simulink model "FunctionalArchitectureProj"  (R2023b)
settings: Solver=VariableStepAuto  StartTime=0.0  StopTime=10.0  RelTol=1e-3
(part 2 of 3)

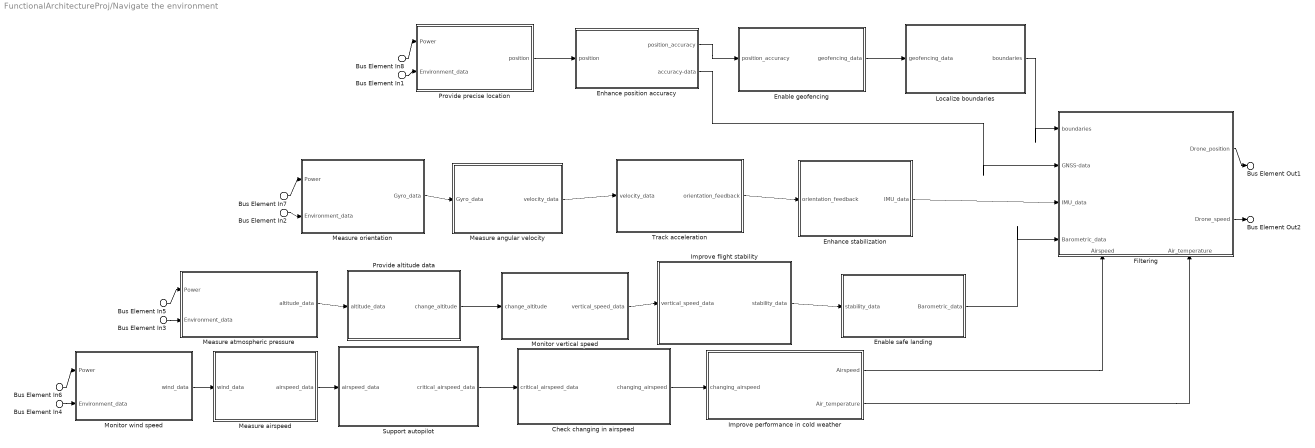
== system FunctionalArchitectureProj/Navigate the environment ==
  Bus Element In{1..4} (4 alike) : Inport  PortName=Environment_data
  Bus Element In{5..8} (4 alike) : Inport  Port=2  PortName=Power
  Check changing in airspeed : Subsystem
      settings: PortSchema="{\"entries\":[{\"content\":{\"headerSize\":26,\"margin\":15,\"minimumSpacing\":25,\"sides\":[{\"content\":{\"connectorIds\":[\"In1\"]},\"type\":\"ConnectorPlacement.EquallySpacedRectSide\",\"uuid\":\"522b493f-2ddf-45ff-a295-a4a6ad43d3e9\"},{\"content\":{\"connectorIds\":[\"Out1\"],\"side\":\"RIGHT\"},\"type\":\"ConnectorPlacement.EquallySpacedRectSide\",\"uuid\":\"9f08b077-98af-4d6e-858b-0cb586e18451\"},{\"content\":{\"side\":\"TOP\"},\"type\":\"ConnectorPlacement.EquallySpacedRectSide\",\"uuid\":\"7ff6f721-17eb-4e7e-8b3a-e93639631da6\"}]},\"type\":\"ConnectorPlacement.EquallySpacedConnector\",\"uuid\":\"bde844eb-2873-40a7-848c-24f407987c7c\"}],\"packageUris\":[\"http://schema.mathworks.com/mf0/Connector/R2020b\"],\"version\":\"1.0\"}"
  Enable geofencing : Subsystem
      settings: PortSchema="{\"entries\":[{\"content\":{\"headerSize\":26,\"margin\":15,\"minimumSpacing\":25,\"sides\":[{\"content\":{\"connectorIds\":[\"In1\"]},\"type\":\"ConnectorPlacement.EquallySpacedRectSide\",\"uuid\":\"522b493f-2ddf-45ff-a295-a4a6ad43d3e9\"},{\"content\":{\"connectorIds\":[\"Out1\"],\"side\":\"RIGHT\"},\"type\":\"ConnectorPlacement.EquallySpacedRectSide\",\"uuid\":\"9f08b077-98af-4d6e-858b-0cb586e18451\"},{\"content\":{\"side\":\"TOP\"},\"type\":\"ConnectorPlacement.EquallySpacedRectSide\",\"uuid\":\"7ff6f721-17eb-4e7e-8b3a-e93639631da6\"}]},\"type\":\"ConnectorPlacement.EquallySpacedConnector\",\"uuid\":\"bde844eb-2873-40a7-848c-24f407987c7c\"}],\"packageUris\":[\"http://schema.mathworks.com/mf0/Connector/R2020b\"],\"version\":\"1.0\"}"
  Enable safe landing : Subsystem
      settings: PortSchema="{\"entries\":[{\"content\":{\"headerSize\":26,\"margin\":15,\"minimumSpacing\":25,\"sides\":[{\"content\":{\"connectorIds\":[\"In1\"]},\"type\":\"ConnectorPlacement.EquallySpacedRectSide\",\"uuid\":\"522b493f-2ddf-45ff-a295-a4a6ad43d3e9\"},{\"content\":{\"connectorIds\":[\"Out1\"],\"side\":\"RIGHT\"},\"type\":\"ConnectorPlacement.EquallySpacedRectSide\",\"uuid\":\"9f08b077-98af-4d6e-858b-0cb586e18451\"},{\"content\":{\"side\":\"TOP\"},\"type\":\"ConnectorPlacement.EquallySpacedRectSide\",\"uuid\":\"7ff6f721-17eb-4e7e-8b3a-e93639631da6\"},{\"content\":{\"side\":\"BOTTOM\"},\"type\":\"ConnectorPlacement.EquallySpacedRectSide\",\"uuid\":\"7f58067e-8efa-428a-9e32-f5196a2d2b76\"}]},\"type\":\"ConnectorPlacement.EquallySpacedConnector\",\"uuid\":\"bde844eb-2873-40a7-848c-24f407987c7c\"}],\"packageUris\":[\"http://schema.mathworks.com/mf0/Connector/R2020b\"],\"version\":\"1.0\"}"
  Enhance position accuracy : Subsystem
      settings: PortSchema="{\"entries\":[{\"content\":{\"headerSize\":26,\"margin\":15,\"minimumSpacing\":25,\"sides\":[{\"content\":{\"connectorIds\":[\"In1\"]},\"type\":\"ConnectorPlacement.EquallySpacedRectSide\",\"uuid\":\"522b493f-2ddf-45ff-a295-a4a6ad43d3e9\"},{\"content\":{\"connectorIds\":[\"Out1\",\"Out2\"],\"side\":\"RIGHT\"},\"type\":\"ConnectorPlacement.EquallySpacedRectSide\",\"uuid\":\"9f08b077-98af-4d6e-858b-0cb586e18451\"},{\"content\":{\"side\":\"TOP\"},\"type\":\"ConnectorPlacement.EquallySpacedRectSide\",\"uuid\":\"7ff6f721-17eb-4e7e-8b3a-e93639631da6\"}]},\"type\":\"ConnectorPlacement.EquallySpacedConnector\",\"uuid\":\"bde844eb-2873-40a7-848c-24f407987c7c\"}],\"packageUris\":[\"http://schema.mathworks.com/mf0/Connector/R2020b\"],\"version\":\"1.0\"}"
  "Enhance stabilization " : Subsystem
      settings: PortSchema="{\"entries\":[{\"content\":{\"headerSize\":26,\"margin\":15,\"minimumSpacing\":25,\"sides\":[{\"content\":{\"connectorIds\":[\"In1\"]},\"type\":\"ConnectorPlacement.EquallySpacedRectSide\",\"uuid\":\"522b493f-2ddf-45ff-a295-a4a6ad43d3e9\"},{\"content\":{\"connectorIds\":[\"Out1\"],\"side\":\"RIGHT\"},\"type\":\"ConnectorPlacement.EquallySpacedRectSide\",\"uuid\":\"9f08b077-98af-4d6e-858b-0cb586e18451\"},{\"content\":{\"side\":\"TOP\"},\"type\":\"ConnectorPlacement.EquallySpacedRectSide\",\"uuid\":\"7ff6f721-17eb-4e7e-8b3a-e93639631da6\"}]},\"type\":\"ConnectorPlacement.EquallySpacedConnector\",\"uuid\":\"bde844eb-2873-40a7-848c-24f407987c7c\"}],\"packageUris\":[\"http://schema.mathworks.com/mf0/Connector/R2020b\"],\"version\":\"1.0\"}"
  Filtering : Subsystem
      settings: PortSchema="{\"entries\":[{\"content\":{\"headerSize\":26,\"margin\":15,\"minimumSpacing\":25,\"sides\":[{\"content\":{\"connectorIds\":[\"In4\",\"In5\",\"In3\",\"In6\"]},\"type\":\"ConnectorPlacement.EquallySpacedRectSide\",\"uuid\":\"522b493f-2ddf-45ff-a295-a4a6ad43d3e9\"},{\"content\":{\"connectorIds\":[\"Out1\",\"Out2\"],\"side\":\"RIGHT\"},\"type\":\"ConnectorPlacement.EquallySpacedRectSide\",\"uuid\":\"9f08b077-98af-4d6e-858b-0cb586e18451\"},{\"content\":{\"side\":\"TOP\"},\"type\":\"ConnectorPlacement.EquallySpacedRectSide\",\"uuid\":\"7ff6f721-17eb-4e7e-8b3a-e93639631da6\"},{\"content\":{\"connectorIds\":[\"In1\",\"In2\"],\"side\":\"BOTTOM\"},\"type\":\"ConnectorPlacement.EquallySpacedRectSide\",\"uuid\":\"1c17908a-7b9e-47dd-bd3a-ac0935137312\"}]},\"type\":\"ConnectorPlacement.EquallySpacedConnector\",\"uuid\":\"bde844eb-2873-40a7-848c-24f407987c7c\"}],\"packageUris\":[\"http://schema.mathworks.com/mf0/Connector/R2020b\"],\"version\":\"1.0\"}"
  Improve flight stability : Subsystem
      settings: PortSchema="{\"entries\":[{\"content\":{\"headerSize\":26,\"margin\":15,\"minimumSpacing\":25,\"sides\":[{\"content\":{\"connectorIds\":[\"In1\"]},\"type\":\"ConnectorPlacement.EquallySpacedRectSide\",\"uuid\":\"522b493f-2ddf-45ff-a295-a4a6ad43d3e9\"},{\"content\":{\"connectorIds\":[\"Out1\"],\"side\":\"RIGHT\"},\"type\":\"ConnectorPlacement.EquallySpacedRectSide\",\"uuid\":\"9f08b077-98af-4d6e-858b-0cb586e18451\"},{\"content\":{\"side\":\"TOP\"},\"type\":\"ConnectorPlacement.EquallySpacedRectSide\",\"uuid\":\"7ff6f721-17eb-4e7e-8b3a-e93639631da6\"}]},\"type\":\"ConnectorPlacement.EquallySpacedConnector\",\"uuid\":\"bde844eb-2873-40a7-848c-24f407987c7c\"}],\"packageUris\":[\"http://schema.mathworks.com/mf0/Connector/R2020b\"],\"version\":\"1.0\"}"
  Improve performance in cold weather : Subsystem
      settings: PortSchema="{\"entries\":[{\"content\":{\"headerSize\":26,\"margin\":15,\"minimumSpacing\":25,\"sides\":[{\"content\":{\"connectorIds\":[\"In1\"]},\"type\":\"ConnectorPlacement.EquallySpacedRectSide\",\"uuid\":\"522b493f-2ddf-45ff-a295-a4a6ad43d3e9\"},{\"content\":{\"connectorIds\":[\"Out1\",\"Out2\"],\"side\":\"RIGHT\"},\"type\":\"ConnectorPlacement.EquallySpacedRectSide\",\"uuid\":\"9f08b077-98af-4d6e-858b-0cb586e18451\"},{\"content\":{\"side\":\"TOP\"},\"type\":\"ConnectorPlacement.EquallySpacedRectSide\",\"uuid\":\"7ff6f721-17eb-4e7e-8b3a-e93639631da6\"}]},\"type\":\"ConnectorPlacement.EquallySpacedConnector\",\"uuid\":\"bde844eb-2873-40a7-848c-24f407987c7c\"}],\"packageUris\":[\"http://schema.mathworks.com/mf0/Connector/R2020b\"],\"version\":\"1.0\"}"
  Localize boundaries : Subsystem
      settings: PortSchema="{\"entries\":[{\"content\":{\"headerSize\":26,\"margin\":15,\"minimumSpacing\":25,\"sides\":[{\"content\":{\"connectorIds\":[\"In1\"]},\"type\":\"ConnectorPlacement.EquallySpacedRectSide\",\"uuid\":\"522b493f-2ddf-45ff-a295-a4a6ad43d3e9\"},{\"content\":{\"connectorIds\":[\"Out1\"],\"side\":\"RIGHT\"},\"type\":\"ConnectorPlacement.EquallySpacedRectSide\",\"uuid\":\"9f08b077-98af-4d6e-858b-0cb586e18451\"},{\"content\":{\"side\":\"TOP\"},\"type\":\"ConnectorPlacement.EquallySpacedRectSide\",\"uuid\":\"7ff6f721-17eb-4e7e-8b3a-e93639631da6\"}]},\"type\":\"ConnectorPlacement.EquallySpacedConnector\",\"uuid\":\"bde844eb-2873-40a7-848c-24f407987c7c\"}],\"packageUris\":[\"http://schema.mathworks.com/mf0/Connector/R2020b\"],\"version\":\"1.0\"}"
  Measure airspeed : Subsystem
      settings: PortSchema="{\"entries\":[{\"content\":{\"headerSize\":26,\"margin\":15,\"minimumSpacing\":25,\"sides\":[{\"content\":{\"connectorIds\":[\"In1\"]},\"type\":\"ConnectorPlacement.EquallySpacedRectSide\",\"uuid\":\"522b493f-2ddf-45ff-a295-a4a6ad43d3e9\"},{\"content\":{\"connectorIds\":[\"Out1\"],\"side\":\"RIGHT\"},\"type\":\"ConnectorPlacement.EquallySpacedRectSide\",\"uuid\":\"9f08b077-98af-4d6e-858b-0cb586e18451\"},{\"content\":{\"side\":\"TOP\"},\"type\":\"ConnectorPlacement.EquallySpacedRectSide\",\"uuid\":\"7ff6f721-17eb-4e7e-8b3a-e93639631da6\"}]},\"type\":\"ConnectorPlacement.EquallySpacedConnector\",\"uuid\":\"bde844eb-2873-40a7-848c-24f407987c7c\"}],\"packageUris\":[\"http://schema.mathworks.com/mf0/Connector/R2020b\"],\"version\":\"1.0\"}"
  Measure angular velocity : Subsystem
      settings: PortSchema="{\"entries\":[{\"content\":{\"headerSize\":26,\"margin\":15,\"minimumSpacing\":25,\"sides\":[{\"content\":{\"connectorIds\":[\"In1\"]},\"type\":\"ConnectorPlacement.EquallySpacedRectSide\",\"uuid\":\"522b493f-2ddf-45ff-a295-a4a6ad43d3e9\"},{\"content\":{\"connectorIds\":[\"Out1\"],\"side\":\"RIGHT\"},\"type\":\"ConnectorPlacement.EquallySpacedRectSide\",\"uuid\":\"9f08b077-98af-4d6e-858b-0cb586e18451\"},{\"content\":{\"side\":\"TOP\"},\"type\":\"ConnectorPlacement.EquallySpacedRectSide\",\"uuid\":\"7ff6f721-17eb-4e7e-8b3a-e93639631da6\"}]},\"type\":\"ConnectorPlacement.EquallySpacedConnector\",\"uuid\":\"bde844eb-2873-40a7-848c-24f407987c7c\"}],\"packageUris\":[\"http://schema.mathworks.com/mf0/Connector/R2020b\"],\"version\":\"1.0\"}"
  Measure atmospheric pressure : Subsystem
      settings: PortSchema="{\"entries\":[{\"content\":{\"headerSize\":26,\"margin\":15,\"minimumSpacing\":25,\"sides\":[{\"content\":{\"connectorIds\":[\"In1\",\"In2\"]},\"type\":\"ConnectorPlacement.EquallySpacedRectSide\",\"uuid\":\"522b493f-2ddf-45ff-a295-a4a6ad43d3e9\"},{\"content\":{\"connectorIds\":[\"Out1\"],\"side\":\"RIGHT\"},\"type\":\"ConnectorPlacement.EquallySpacedRectSide\",\"uuid\":\"9f08b077-98af-4d6e-858b-0cb586e18451\"},{\"content\":{\"side\":\"TOP\"},\"type\":\"ConnectorPlacement.EquallySpacedRectSide\",\"uuid\":\"7ff6f721-17eb-4e7e-8b3a-e93639631da6\"}]},\"type\":\"ConnectorPlacement.EquallySpacedConnector\",\"uuid\":\"bde844eb-2873-40a7-848c-24f407987c7c\"}],\"packageUris\":[\"http://schema.mathworks.com/mf0/Connector/R2020b\"],\"version\":\"1.0\"}"
  Measure orientation : Subsystem
      settings: PortSchema="{\"entries\":[{\"content\":{\"headerSize\":26,\"margin\":15,\"minimumSpacing\":25,\"sides\":[{\"content\":{\"connectorIds\":[\"In1\",\"In2\"]},\"type\":\"ConnectorPlacement.EquallySpacedRectSide\",\"uuid\":\"522b493f-2ddf-45ff-a295-a4a6ad43d3e9\"},{\"content\":{\"connectorIds\":[\"Out1\"],\"side\":\"RIGHT\"},\"type\":\"ConnectorPlacement.EquallySpacedRectSide\",\"uuid\":\"9f08b077-98af-4d6e-858b-0cb586e18451\"},{\"content\":{\"side\":\"TOP\"},\"type\":\"ConnectorPlacement.EquallySpacedRectSide\",\"uuid\":\"7ff6f721-17eb-4e7e-8b3a-e93639631da6\"}]},\"type\":\"ConnectorPlacement.EquallySpacedConnector\",\"uuid\":\"bde844eb-2873-40a7-848c-24f407987c7c\"}],\"packageUris\":[\"http://schema.mathworks.com/mf0/Connector/R2020b\"],\"version\":\"1.0\"}"
  Monitor vertical speed : Subsystem
      settings: PortSchema="{\"entries\":[{\"content\":{\"headerSize\":26,\"margin\":15,\"minimumSpacing\":25,\"sides\":[{\"content\":{\"connectorIds\":[\"In1\"]},\"type\":\"ConnectorPlacement.EquallySpacedRectSide\",\"uuid\":\"522b493f-2ddf-45ff-a295-a4a6ad43d3e9\"},{\"content\":{\"connectorIds\":[\"Out1\"],\"side\":\"RIGHT\"},\"type\":\"ConnectorPlacement.EquallySpacedRectSide\",\"uuid\":\"9f08b077-98af-4d6e-858b-0cb586e18451\"},{\"content\":{\"side\":\"TOP\"},\"type\":\"ConnectorPlacement.EquallySpacedRectSide\",\"uuid\":\"7ff6f721-17eb-4e7e-8b3a-e93639631da6\"}]},\"type\":\"ConnectorPlacement.EquallySpacedConnector\",\"uuid\":\"bde844eb-2873-40a7-848c-24f407987c7c\"}],\"packageUris\":[\"http://schema.mathworks.com/mf0/Connector/R2020b\"],\"version\":\"1.0\"}"
  Monitor wind speed : Subsystem
      settings: PortSchema="{\"entries\":[{\"content\":{\"headerSize\":26,\"margin\":15,\"minimumSpacing\":25,\"sides\":[{\"content\":{\"connectorIds\":[\"In1\",\"In2\"]},\"type\":\"ConnectorPlacement.EquallySpacedRectSide\",\"uuid\":\"522b493f-2ddf-45ff-a295-a4a6ad43d3e9\"},{\"content\":{\"connectorIds\":[\"Out1\"],\"side\":\"RIGHT\"},\"type\":\"ConnectorPlacement.EquallySpacedRectSide\",\"uuid\":\"9f08b077-98af-4d6e-858b-0cb586e18451\"},{\"content\":{\"side\":\"TOP\"},\"type\":\"ConnectorPlacement.EquallySpacedRectSide\",\"uuid\":\"7ff6f721-17eb-4e7e-8b3a-e93639631da6\"}]},\"type\":\"ConnectorPlacement.EquallySpacedConnector\",\"uuid\":\"bde844eb-2873-40a7-848c-24f407987c7c\"}],\"packageUris\":[\"http://schema.mathworks.com/mf0/Connector/R2020b\"],\"version\":\"1.0\"}"
  Provide altitude data : Subsystem
      settings: PortSchema="{\"entries\":[{\"content\":{\"headerSize\":26,\"margin\":15,\"minimumSpacing\":25,\"sides\":[{\"content\":{\"connectorIds\":[\"In1\"]},\"type\":\"ConnectorPlacement.EquallySpacedRectSide\",\"uuid\":\"522b493f-2ddf-45ff-a295-a4a6ad43d3e9\"},{\"content\":{\"connectorIds\":[\"Out1\"],\"side\":\"RIGHT\"},\"type\":\"ConnectorPlacement.EquallySpacedRectSide\",\"uuid\":\"9f08b077-98af-4d6e-858b-0cb586e18451\"},{\"content\":{\"side\":\"TOP\"},\"type\":\"ConnectorPlacement.EquallySpacedRectSide\",\"uuid\":\"7ff6f721-17eb-4e7e-8b3a-e93639631da6\"}]},\"type\":\"ConnectorPlacement.EquallySpacedConnector\",\"uuid\":\"bde844eb-2873-40a7-848c-24f407987c7c\"}],\"packageUris\":[\"http://schema.mathworks.com/mf0/Connector/R2020b\"],\"version\":\"1.0\"}"
  Provide precise location : Subsystem
      settings: PortSchema="{\"entries\":[{\"content\":{\"headerSize\":26,\"margin\":15,\"minimumSpacing\":25,\"sides\":[{\"content\":{\"connectorIds\":[\"In1\",\"In2\"]},\"type\":\"ConnectorPlacement.EquallySpacedRectSide\",\"uuid\":\"522b493f-2ddf-45ff-a295-a4a6ad43d3e9\"},{\"content\":{\"connectorIds\":[\"Out1\"],\"side\":\"RIGHT\"},\"type\":\"ConnectorPlacement.EquallySpacedRectSide\",\"uuid\":\"9f08b077-98af-4d6e-858b-0cb586e18451\"},{\"content\":{\"side\":\"TOP\"},\"type\":\"ConnectorPlacement.EquallySpacedRectSide\",\"uuid\":\"7ff6f721-17eb-4e7e-8b3a-e93639631da6\"}]},\"type\":\"ConnectorPlacement.EquallySpacedConnector\",\"uuid\":\"bde844eb-2873-40a7-848c-24f407987c7c\"}],\"packageUris\":[\"http://schema.mathworks.com/mf0/Connector/R2020b\"],\"version\":\"1.0\"}"
  Support autopilot : Subsystem
      settings: PortSchema="{\"entries\":[{\"content\":{\"headerSize\":26,\"margin\":15,\"minimumSpacing\":25,\"sides\":[{\"content\":{\"connectorIds\":[\"In1\"]},\"type\":\"ConnectorPlacement.EquallySpacedRectSide\",\"uuid\":\"522b493f-2ddf-45ff-a295-a4a6ad43d3e9\"},{\"content\":{\"connectorIds\":[\"Out1\"],\"side\":\"RIGHT\"},\"type\":\"ConnectorPlacement.EquallySpacedRectSide\",\"uuid\":\"9f08b077-98af-4d6e-858b-0cb586e18451\"},{\"content\":{\"side\":\"TOP\"},\"type\":\"ConnectorPlacement.EquallySpacedRectSide\",\"uuid\":\"7ff6f721-17eb-4e7e-8b3a-e93639631da6\"}]},\"type\":\"ConnectorPlacement.EquallySpacedConnector\",\"uuid\":\"bde844eb-2873-40a7-848c-24f407987c7c\"}],\"packageUris\":[\"http://schema.mathworks.com/mf0/Connector/R2020b\"],\"version\":\"1.0\"}"
  Track acceleration : Subsystem
      settings: PortSchema="{\"entries\":[{\"content\":{\"headerSize\":26,\"margin\":15,\"minimumSpacing\":25,\"sides\":[{\"content\":{\"connectorIds\":[\"In1\"]},\"type\":\"ConnectorPlacement.EquallySpacedRectSide\",\"uuid\":\"522b493f-2ddf-45ff-a295-a4a6ad43d3e9\"},{\"content\":{\"connectorIds\":[\"Out1\"],\"side\":\"RIGHT\"},\"type\":\"ConnectorPlacement.EquallySpacedRectSide\",\"uuid\":\"9f08b077-98af-4d6e-858b-0cb586e18451\"},{\"content\":{\"side\":\"TOP\"},\"type\":\"ConnectorPlacement.EquallySpacedRectSide\",\"uuid\":\"7ff6f721-17eb-4e7e-8b3a-e93639631da6\"}]},\"type\":\"ConnectorPlacement.EquallySpacedConnector\",\"uuid\":\"bde844eb-2873-40a7-848c-24f407987c7c\"}],\"packageUris\":[\"http://schema.mathworks.com/mf0/Connector/R2020b\"],\"version\":\"1.0\"}"
  Bus Element Out1 : Outport  PortName=Drone_position
  Bus Element Out2 : Outport  Port=2  PortName=Drone_speed
  wires:
  Provide precise location/1(position) -> Enhance position accuracy/1(position)
  Enhance position accuracy/1(position_accuracy) -> Enable geofencing/1(position_accuracy)
  Enable geofencing/1(geofencing_data) -> Localize boundaries/1(geofencing_data)
  Enhance position accuracy/2(accuracy-data) -> Filtering/5(GNSS-data)
  Measure orientation/1(Gyro_data) -> Measure angular velocity/1(Gyro_data)
  Localize boundaries/1(boundaries) -> Filtering/4(boundaries)
  Track acceleration/1(orientation_feedback) -> "Enhance stabilization "/1(orientation_feedback)
  Measure angular velocity/1(velocity_data) -> Track acceleration/1(velocity_data)
  "Enhance stabilization "/1(IMU_data) -> Filtering/3(IMU_data)
  Measure atmospheric pressure/1(altitude_data) -> Provide altitude data/1(altitude_data)
  Enable safe landing/1(Barometric_data) -> Filtering/6(Barometric_data)
  Provide altitude data/1(change_altitude) -> Monitor vertical speed/1(change_altitude)
  Monitor vertical speed/1(vertical_speed_data) -> Improve flight stability/1(vertical_speed_data)
  Improve flight stability/1(stability_data) -> Enable safe landing/1(stability_data)
  Monitor wind speed/1(wind_data) -> Measure airspeed/1(wind_data)
  Measure airspeed/1(airspeed_data) -> Support autopilot/1(airspeed_data)
  Support autopilot/1(critical_airspeed_data) -> Check changing in airspeed/1(critical_airspeed_data)
  Check changing in airspeed/1(changing_airspeed) -> Improve performance in cold weather/1(changing_airspeed)
  Improve performance in cold weather/1(Airspeed) -> Filtering/1(Airspeed)
  Improve performance in cold weather/2(Air_temperature) -> Filtering/2(Air_temperature)
  Bus Element In1/1 -> Provide precise location/2(Environment_data)
  Bus Element In2/1 -> Measure orientation/2(Environment_data)
  Bus Element In3/1 -> Measure atmospheric pressure/2(Environment_data)
  Bus Element In4/1 -> Monitor wind speed/2(Environment_data)
  Filtering/1(Drone_position) -> Bus Element Out1/1
  Filtering/2(Drone_speed) -> Bus Element Out2/1
  Bus Element In5/1 -> Measure atmospheric pressure/1(Power)
  Bus Element In6/1 -> Monitor wind speed/1(Power)
  Bus Element In7/1 -> Measure orientation/1(Power)
  Bus Element In8/1 -> Provide precise location/1(Power)

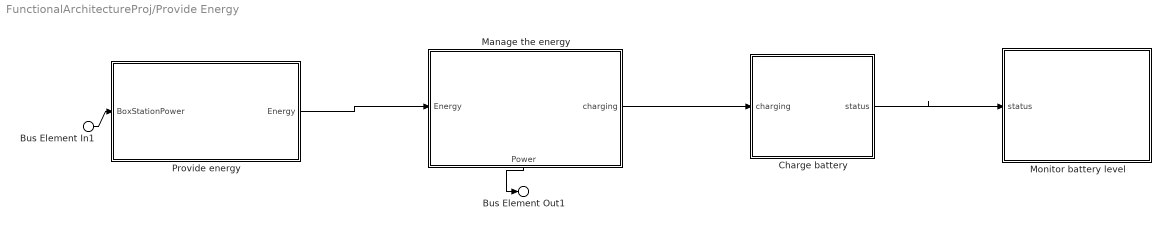
== system FunctionalArchitectureProj/Provide Energy ==
  Bus Element In1 : Inport  PortName=BoxStationPower
  Charge battery : Subsystem
      settings: PortSchema="{\"entries\":[{\"content\":{\"headerSize\":26,\"margin\":15,\"minimumSpacing\":25,\"sides\":[{\"content\":{\"connectorIds\":[\"In1\"]},\"type\":\"ConnectorPlacement.EquallySpacedRectSide\",\"uuid\":\"9cca9539-0a36-4124-b22c-ee31f3591a67\"},{\"content\":{\"connectorIds\":[\"Out1\"],\"side\":\"RIGHT\"},\"type\":\"ConnectorPlacement.EquallySpacedRectSide\",\"uuid\":\"eebe1ec1-c849-468b-8863-53f0cc841d23\"},{\"content\":{\"side\":\"TOP\"},\"type\":\"ConnectorPlacement.EquallySpacedRectSide\",\"uuid\":\"8f1c4dda-9d7f-4fb5-99d0-4e96ed432329\"}]},\"type\":\"ConnectorPlacement.EquallySpacedConnector\",\"uuid\":\"f7d57f3a-667c-4dfa-8f30-8433699dfbc6\"}],\"packageUris\":[\"http://schema.mathworks.com/mf0/Connector/R2020b\"],\"version\":\"1.0\"}"
  Manage the energy : Subsystem
      settings: PortSchema="{\"entries\":[{\"content\":{\"headerSize\":26,\"margin\":15,\"minimumSpacing\":25,\"sides\":[{\"content\":{\"connectorIds\":[\"In1\"]},\"type\":\"ConnectorPlacement.EquallySpacedRectSide\",\"uuid\":\"c0b5e0bb-d2bf-4d40-b1ad-0d63f5f2311e\"},{\"content\":{\"connectorIds\":[\"Out2\"],\"side\":\"RIGHT\"},\"type\":\"ConnectorPlacement.EquallySpacedRectSide\",\"uuid\":\"73104a81-7012-49ca-8030-68cbb7243dfa\"},{\"content\":{\"side\":\"TOP\"},\"type\":\"ConnectorPlacement.EquallySpacedRectSide\",\"uuid\":\"7c311739-eaa1-403c-a576-4458554363b2\"},{\"content\":{\"connectorIds\":[\"Out1\"],\"side\":\"BOTTOM\"},\"type\":\"ConnectorPlacement.EquallySpacedRectSide\",\"uuid\":\"6353551f-44ff-4ee3-b4c3-711b036adab5\"}]},\"type\":\"ConnectorPlacement.EquallySpacedConnector\",\"uuid\":\"83a80a93-0958-4176-98e5-b02d609066aa\"}],\"packageUris\":[\"http://schema.mathworks.com/mf0/Connector/R2020b\"],\"version\":\"1.0\"}"
  Monitor battery level : Subsystem
      settings: PortSchema="{\"entries\":[{\"content\":{\"headerSize\":26,\"margin\":15,\"minimumSpacing\":25,\"sides\":[{\"content\":{\"connectorIds\":[\"In1\"]},\"type\":\"ConnectorPlacement.EquallySpacedRectSide\",\"uuid\":\"9cca9539-0a36-4124-b22c-ee31f3591a67\"},{\"content\":{\"side\":\"RIGHT\"},\"type\":\"ConnectorPlacement.EquallySpacedRectSide\",\"uuid\":\"eebe1ec1-c849-468b-8863-53f0cc841d23\"},{\"content\":{\"side\":\"TOP\"},\"type\":\"ConnectorPlacement.EquallySpacedRectSide\",\"uuid\":\"8f1c4dda-9d7f-4fb5-99d0-4e96ed432329\"}]},\"type\":\"ConnectorPlacement.EquallySpacedConnector\",\"uuid\":\"f7d57f3a-667c-4dfa-8f30-8433699dfbc6\"}],\"packageUris\":[\"http://schema.mathworks.com/mf0/Connector/R2020b\"],\"version\":\"1.0\"}"
  "Provide energy " : Subsystem
      settings: PortSchema="{\"entries\":[{\"content\":{\"headerSize\":26,\"margin\":15,\"minimumSpacing\":25,\"sides\":[{\"content\":{\"connectorIds\":[\"In1\"]},\"type\":\"ConnectorPlacement.EquallySpacedRectSide\",\"uuid\":\"9cca9539-0a36-4124-b22c-ee31f3591a67\"},{\"content\":{\"connectorIds\":[\"Out1\"],\"side\":\"RIGHT\"},\"type\":\"ConnectorPlacement.EquallySpacedRectSide\",\"uuid\":\"eebe1ec1-c849-468b-8863-53f0cc841d23\"},{\"content\":{\"side\":\"TOP\"},\"type\":\"ConnectorPlacement.EquallySpacedRectSide\",\"uuid\":\"8f1c4dda-9d7f-4fb5-99d0-4e96ed432329\"}]},\"type\":\"ConnectorPlacement.EquallySpacedConnector\",\"uuid\":\"f7d57f3a-667c-4dfa-8f30-8433699dfbc6\"}],\"packageUris\":[\"http://schema.mathworks.com/mf0/Connector/R2020b\"],\"version\":\"1.0\"}"
  Bus Element Out1 : Outport  PortName=Power
  wires:
  "Provide energy "/1(Energy) -> Manage the energy/1(Energy)
  Manage the energy/2(charging) -> Charge battery/1(charging)
  Charge battery/1(status) -> Monitor battery level/1(status)
  Manage the energy/1(Power) -> Bus Element Out1/1
  Bus Element In1/1 -> "Provide energy "/1(BoxStationPower)

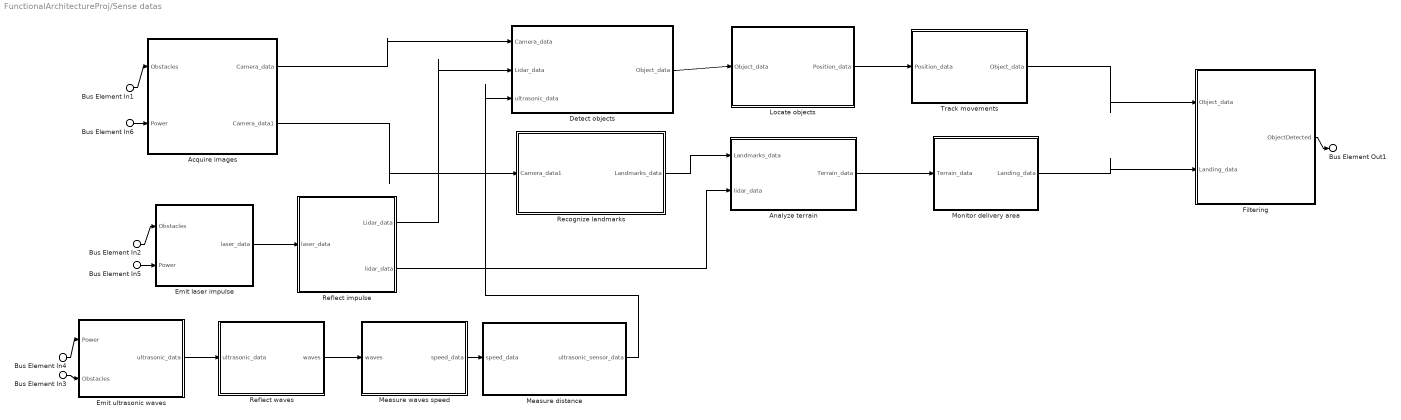
== system FunctionalArchitectureProj/Sense datas ==
  Bus Element In1 : Inport  PortName=Obstacles
  Bus Element In2 : Inport  PortName=Obstacles
  Bus Element In3 : Inport  PortName=Obstacles
  Bus Element In4 : Inport  Port=2  PortName=Power
  Bus Element In5 : Inport  Port=2  PortName=Power
  Bus Element In6 : Inport  Port=2  PortName=Power
  Acquire images : Subsystem
      settings: PortSchema="{\"entries\":[{\"content\":{\"headerSize\":26,\"margin\":15,\"minimumSpacing\":25,\"sides\":[{\"content\":{\"connectorIds\":[\"In1\",\"In2\"]},\"type\":\"ConnectorPlacement.EquallySpacedRectSide\",\"uuid\":\"c0b5e0bb-d2bf-4d40-b1ad-0d63f5f2311e\"},{\"content\":{\"connectorIds\":[\"Out1\",\"Out2\"],\"side\":\"RIGHT\"},\"type\":\"ConnectorPlacement.EquallySpacedRectSide\",\"uuid\":\"73104a81-7012-49ca-8030-68cbb7243dfa\"},{\"content\":{\"side\":\"TOP\"},\"type\":\"ConnectorPlacement.EquallySpacedRectSide\",\"uuid\":\"7c311739-eaa1-403c-a576-4458554363b2\"}]},\"type\":\"ConnectorPlacement.EquallySpacedConnector\",\"uuid\":\"83a80a93-0958-4176-98e5-b02d609066aa\"}],\"packageUris\":[\"http://schema.mathworks.com/mf0/Connector/R2020b\"],\"version\":\"1.0\"}"
  Analyze terrain : Subsystem
      settings: PortSchema="{\"entries\":[{\"content\":{\"headerSize\":26,\"margin\":15,\"minimumSpacing\":25,\"sides\":[{\"content\":{\"connectorIds\":[\"In1\",\"In2\"]},\"type\":\"ConnectorPlacement.EquallySpacedRectSide\",\"uuid\":\"522b493f-2ddf-45ff-a295-a4a6ad43d3e9\"},{\"content\":{\"connectorIds\":[\"Out1\"],\"side\":\"RIGHT\"},\"type\":\"ConnectorPlacement.EquallySpacedRectSide\",\"uuid\":\"9f08b077-98af-4d6e-858b-0cb586e18451\"},{\"content\":{\"side\":\"TOP\"},\"type\":\"ConnectorPlacement.EquallySpacedRectSide\",\"uuid\":\"7ff6f721-17eb-4e7e-8b3a-e93639631da6\"}]},\"type\":\"ConnectorPlacement.EquallySpacedConnector\",\"uuid\":\"bde844eb-2873-40a7-848c-24f407987c7c\"}],\"packageUris\":[\"http://schema.mathworks.com/mf0/Connector/R2020b\"],\"version\":\"1.0\"}"
  Detect objects : Subsystem
      settings: PortSchema="{\"entries\":[{\"content\":{\"headerSize\":26,\"margin\":15,\"minimumSpacing\":25,\"sides\":[{\"content\":{\"connectorIds\":[\"In1\",\"In2\",\"In3\"]},\"type\":\"ConnectorPlacement.EquallySpacedRectSide\",\"uuid\":\"c0b5e0bb-d2bf-4d40-b1ad-0d63f5f2311e\"},{\"content\":{\"connectorIds\":[\"Out1\"],\"side\":\"RIGHT\"},\"type\":\"ConnectorPlacement.EquallySpacedRectSide\",\"uuid\":\"73104a81-7012-49ca-8030-68cbb7243dfa\"},{\"content\":{\"side\":\"TOP\"},\"type\":\"ConnectorPlacement.EquallySpacedRectSide\",\"uuid\":\"7c311739-eaa1-403c-a576-4458554363b2\"}]},\"type\":\"ConnectorPlacement.EquallySpacedConnector\",\"uuid\":\"83a80a93-0958-4176-98e5-b02d609066aa\"}],\"packageUris\":[\"http://schema.mathworks.com/mf0/Connector/R2020b\"],\"version\":\"1.0\"}"
  Emit laser impulse : Subsystem
      settings: PortSchema="{\"entries\":[{\"content\":{\"headerSize\":26,\"margin\":15,\"minimumSpacing\":25,\"sides\":[{\"content\":{\"connectorIds\":[\"In1\",\"In2\"]},\"type\":\"ConnectorPlacement.EquallySpacedRectSide\",\"uuid\":\"c0b5e0bb-d2bf-4d40-b1ad-0d63f5f2311e\"},{\"content\":{\"connectorIds\":[\"Out1\"],\"side\":\"RIGHT\"},\"type\":\"ConnectorPlacement.EquallySpacedRectSide\",\"uuid\":\"73104a81-7012-49ca-8030-68cbb7243dfa\"},{\"content\":{\"side\":\"TOP\"},\"type\":\"ConnectorPlacement.EquallySpacedRectSide\",\"uuid\":\"7c311739-eaa1-403c-a576-4458554363b2\"},{\"content\":{\"side\":\"BOTTOM\"},\"type\":\"ConnectorPlacement.EquallySpacedRectSide\",\"uuid\":\"1fdf15b1-8a8d-4350-bda7-0c86e31633d1\"}]},\"type\":\"ConnectorPlacement.EquallySpacedConnector\",\"uuid\":\"83a80a93-0958-4176-98e5-b02d609066aa\"}],\"packageUris\":[\"http://schema.mathworks.com/mf0/Connector/R2020b\"],\"version\":\"1.0\"}"
  Emit ultrasonic waves : Subsystem
      settings: PortSchema="{\"entries\":[{\"content\":{\"headerSize\":26,\"margin\":15,\"minimumSpacing\":25,\"sides\":[{\"content\":{\"connectorIds\":[\"In1\",\"In2\"]},\"type\":\"ConnectorPlacement.EquallySpacedRectSide\",\"uuid\":\"522b493f-2ddf-45ff-a295-a4a6ad43d3e9\"},{\"content\":{\"connectorIds\":[\"Out1\"],\"side\":\"RIGHT\"},\"type\":\"ConnectorPlacement.EquallySpacedRectSide\",\"uuid\":\"9f08b077-98af-4d6e-858b-0cb586e18451\"},{\"content\":{\"side\":\"TOP\"},\"type\":\"ConnectorPlacement.EquallySpacedRectSide\",\"uuid\":\"7ff6f721-17eb-4e7e-8b3a-e93639631da6\"}]},\"type\":\"ConnectorPlacement.EquallySpacedConnector\",\"uuid\":\"bde844eb-2873-40a7-848c-24f407987c7c\"}],\"packageUris\":[\"http://schema.mathworks.com/mf0/Connector/R2020b\"],\"version\":\"1.0\"}"
  Filtering : Subsystem
      settings: PortSchema="{\"entries\":[{\"content\":{\"headerSize\":26,\"margin\":15,\"minimumSpacing\":25,\"sides\":[{\"content\":{\"connectorIds\":[\"In1\",\"In2\"]},\"type\":\"ConnectorPlacement.EquallySpacedRectSide\",\"uuid\":\"9cca9539-0a36-4124-b22c-ee31f3591a67\"},{\"content\":{\"connectorIds\":[\"Out1\"],\"side\":\"RIGHT\"},\"type\":\"ConnectorPlacement.EquallySpacedRectSide\",\"uuid\":\"eebe1ec1-c849-468b-8863-53f0cc841d23\"},{\"content\":{\"side\":\"TOP\"},\"type\":\"ConnectorPlacement.EquallySpacedRectSide\",\"uuid\":\"8f1c4dda-9d7f-4fb5-99d0-4e96ed432329\"}]},\"type\":\"ConnectorPlacement.EquallySpacedConnector\",\"uuid\":\"f7d57f3a-667c-4dfa-8f30-8433699dfbc6\"}],\"packageUris\":[\"http://schema.mathworks.com/mf0/Connector/R2020b\"],\"version\":\"1.0\"}"
  Locate objects : Subsystem
      settings: PortSchema="{\"entries\":[{\"content\":{\"headerSize\":26,\"margin\":15,\"minimumSpacing\":25,\"sides\":[{\"content\":{\"connectorIds\":[\"In1\"]},\"type\":\"ConnectorPlacement.EquallySpacedRectSide\",\"uuid\":\"522b493f-2ddf-45ff-a295-a4a6ad43d3e9\"},{\"content\":{\"connectorIds\":[\"Out1\"],\"side\":\"RIGHT\"},\"type\":\"ConnectorPlacement.EquallySpacedRectSide\",\"uuid\":\"9f08b077-98af-4d6e-858b-0cb586e18451\"},{\"content\":{\"side\":\"TOP\"},\"type\":\"ConnectorPlacement.EquallySpacedRectSide\",\"uuid\":\"7ff6f721-17eb-4e7e-8b3a-e93639631da6\"}]},\"type\":\"ConnectorPlacement.EquallySpacedConnector\",\"uuid\":\"bde844eb-2873-40a7-848c-24f407987c7c\"}],\"packageUris\":[\"http://schema.mathworks.com/mf0/Connector/R2020b\"],\"version\":\"1.0\"}"
  Measure distance : Subsystem
      settings: PortSchema="{\"entries\":[{\"content\":{\"headerSize\":26,\"margin\":15,\"minimumSpacing\":25,\"sides\":[{\"content\":{\"connectorIds\":[\"In1\"]},\"type\":\"ConnectorPlacement.EquallySpacedRectSide\",\"uuid\":\"522b493f-2ddf-45ff-a295-a4a6ad43d3e9\"},{\"content\":{\"connectorIds\":[\"Out1\"],\"side\":\"RIGHT\"},\"type\":\"ConnectorPlacement.EquallySpacedRectSide\",\"uuid\":\"9f08b077-98af-4d6e-858b-0cb586e18451\"},{\"content\":{\"side\":\"TOP\"},\"type\":\"ConnectorPlacement.EquallySpacedRectSide\",\"uuid\":\"7ff6f721-17eb-4e7e-8b3a-e93639631da6\"}]},\"type\":\"ConnectorPlacement.EquallySpacedConnector\",\"uuid\":\"bde844eb-2873-40a7-848c-24f407987c7c\"}],\"packageUris\":[\"http://schema.mathworks.com/mf0/Connector/R2020b\"],\"version\":\"1.0\"}"
  Measure waves speed : Subsystem
      settings: PortSchema="{\"entries\":[{\"content\":{\"headerSize\":26,\"margin\":15,\"minimumSpacing\":25,\"sides\":[{\"content\":{\"connectorIds\":[\"In1\"]},\"type\":\"ConnectorPlacement.EquallySpacedRectSide\",\"uuid\":\"522b493f-2ddf-45ff-a295-a4a6ad43d3e9\"},{\"content\":{\"connectorIds\":[\"Out1\"],\"side\":\"RIGHT\"},\"type\":\"ConnectorPlacement.EquallySpacedRectSide\",\"uuid\":\"9f08b077-98af-4d6e-858b-0cb586e18451\"},{\"content\":{\"side\":\"TOP\"},\"type\":\"ConnectorPlacement.EquallySpacedRectSide\",\"uuid\":\"7ff6f721-17eb-4e7e-8b3a-e93639631da6\"}]},\"type\":\"ConnectorPlacement.EquallySpacedConnector\",\"uuid\":\"bde844eb-2873-40a7-848c-24f407987c7c\"}],\"packageUris\":[\"http://schema.mathworks.com/mf0/Connector/R2020b\"],\"version\":\"1.0\"}"
  Monitor delivery area : Subsystem
      settings: PortSchema="{\"entries\":[{\"content\":{\"headerSize\":26,\"margin\":15,\"minimumSpacing\":25,\"sides\":[{\"content\":{\"connectorIds\":[\"In1\"]},\"type\":\"ConnectorPlacement.EquallySpacedRectSide\",\"uuid\":\"522b493f-2ddf-45ff-a295-a4a6ad43d3e9\"},{\"content\":{\"connectorIds\":[\"Out1\"],\"side\":\"RIGHT\"},\"type\":\"ConnectorPlacement.EquallySpacedRectSide\",\"uuid\":\"9f08b077-98af-4d6e-858b-0cb586e18451\"},{\"content\":{\"side\":\"TOP\"},\"type\":\"ConnectorPlacement.EquallySpacedRectSide\",\"uuid\":\"7ff6f721-17eb-4e7e-8b3a-e93639631da6\"},{\"content\":{\"side\":\"BOTTOM\"},\"type\":\"ConnectorPlacement.EquallySpacedRectSide\",\"uuid\":\"db146416-0b47-4dd0-b7bf-6933d884648d\"}]},\"type\":\"ConnectorPlacement.EquallySpacedConnector\",\"uuid\":\"bde844eb-2873-40a7-848c-24f407987c7c\"}],\"packageUris\":[\"http://schema.mathworks.com/mf0/Connector/R2020b\"],\"version\":\"1.0\"}"
  Recognize landmarks : Subsystem
      settings: PortSchema="{\"entries\":[{\"content\":{\"headerSize\":26,\"margin\":15,\"minimumSpacing\":25,\"sides\":[{\"content\":{\"connectorIds\":[\"In1\"]},\"type\":\"ConnectorPlacement.EquallySpacedRectSide\",\"uuid\":\"c0b5e0bb-d2bf-4d40-b1ad-0d63f5f2311e\"},{\"content\":{\"connectorIds\":[\"Out1\"],\"side\":\"RIGHT\"},\"type\":\"ConnectorPlacement.EquallySpacedRectSide\",\"uuid\":\"73104a81-7012-49ca-8030-68cbb7243dfa\"},{\"content\":{\"side\":\"TOP\"},\"type\":\"ConnectorPlacement.EquallySpacedRectSide\",\"uuid\":\"7c311739-eaa1-403c-a576-4458554363b2\"}]},\"type\":\"ConnectorPlacement.EquallySpacedConnector\",\"uuid\":\"83a80a93-0958-4176-98e5-b02d609066aa\"}],\"packageUris\":[\"http://schema.mathworks.com/mf0/Connector/R2020b\"],\"version\":\"1.0\"}"
  Reflect impulse : Subsystem
      settings: PortSchema="{\"entries\":[{\"content\":{\"headerSize\":26,\"margin\":15,\"minimumSpacing\":25,\"sides\":[{\"content\":{\"connectorIds\":[\"In1\"]},\"type\":\"ConnectorPlacement.EquallySpacedRectSide\",\"uuid\":\"c0b5e0bb-d2bf-4d40-b1ad-0d63f5f2311e\"},{\"content\":{\"connectorIds\":[\"Out1\",\"Out2\"],\"side\":\"RIGHT\"},\"type\":\"ConnectorPlacement.EquallySpacedRectSide\",\"uuid\":\"73104a81-7012-49ca-8030-68cbb7243dfa\"},{\"content\":{\"side\":\"TOP\"},\"type\":\"ConnectorPlacement.EquallySpacedRectSide\",\"uuid\":\"7c311739-eaa1-403c-a576-4458554363b2\"}]},\"type\":\"ConnectorPlacement.EquallySpacedConnector\",\"uuid\":\"83a80a93-0958-4176-98e5-b02d609066aa\"}],\"packageUris\":[\"http://schema.mathworks.com/mf0/Connector/R2020b\"],\"version\":\"1.0\"}"
  Reflect waves : Subsystem
      settings: PortSchema="{\"entries\":[{\"content\":{\"headerSize\":26,\"margin\":15,\"minimumSpacing\":25,\"sides\":[{\"content\":{\"connectorIds\":[\"In1\"]},\"type\":\"ConnectorPlacement.EquallySpacedRectSide\",\"uuid\":\"522b493f-2ddf-45ff-a295-a4a6ad43d3e9\"},{\"content\":{\"connectorIds\":[\"Out1\"],\"side\":\"RIGHT\"},\"type\":\"ConnectorPlacement.EquallySpacedRectSide\",\"uuid\":\"9f08b077-98af-4d6e-858b-0cb586e18451\"},{\"content\":{\"side\":\"TOP\"},\"type\":\"ConnectorPlacement.EquallySpacedRectSide\",\"uuid\":\"7ff6f721-17eb-4e7e-8b3a-e93639631da6\"}]},\"type\":\"ConnectorPlacement.EquallySpacedConnector\",\"uuid\":\"bde844eb-2873-40a7-848c-24f407987c7c\"}],\"packageUris\":[\"http://schema.mathworks.com/mf0/Connector/R2020b\"],\"version\":\"1.0\"}"
  Track movements : Subsystem
      settings: PortSchema="{\"entries\":[{\"content\":{\"headerSize\":26,\"margin\":15,\"minimumSpacing\":25,\"sides\":[{\"content\":{\"connectorIds\":[\"In1\"]},\"type\":\"ConnectorPlacement.EquallySpacedRectSide\",\"uuid\":\"522b493f-2ddf-45ff-a295-a4a6ad43d3e9\"},{\"content\":{\"connectorIds\":[\"Out1\"],\"side\":\"RIGHT\"},\"type\":\"ConnectorPlacement.EquallySpacedRectSide\",\"uuid\":\"9f08b077-98af-4d6e-858b-0cb586e18451\"},{\"content\":{\"side\":\"TOP\"},\"type\":\"ConnectorPlacement.EquallySpacedRectSide\",\"uuid\":\"7ff6f721-17eb-4e7e-8b3a-e93639631da6\"}]},\"type\":\"ConnectorPlacement.EquallySpacedConnector\",\"uuid\":\"bde844eb-2873-40a7-848c-24f407987c7c\"}],\"packageUris\":[\"http://schema.mathworks.com/mf0/Connector/R2020b\"],\"version\":\"1.0\"}"
  Bus Element Out1 : Outport  PortName=ObjectDetected
  wires:
  Emit laser impulse/1(laser_data) -> Reflect impulse/1(laser_data)
  Acquire images/1(Camera_data) -> Detect objects/1(Camera_data)
  Acquire images/2(Camera_data1) -> Recognize landmarks/1(Camera_data1)
  Track movements/1(Object_data) -> Filtering/1(Object_data)
  Detect objects/1(Object_data) -> Locate objects/1(Object_data)
  Recognize landmarks/1(Landmarks_data) -> Analyze terrain/1(Landmarks_data)
  Locate objects/1(Position_data) -> Track movements/1(Position_data)
  Analyze terrain/1(Terrain_data) -> Monitor delivery area/1(Terrain_data)
  Reflect impulse/1(Lidar_data) -> Detect objects/2(Lidar_data)
  Reflect impulse/2(lidar_data) -> Analyze terrain/2(lidar_data)
  Monitor delivery area/1(Landing_data) -> Filtering/2(Landing_data)
  Emit ultrasonic waves/1(ultrasonic_data) -> Reflect waves/1(ultrasonic_data)
  Reflect waves/1(waves) -> Measure waves speed/1(waves)
  Measure waves speed/1(speed_data) -> Measure distance/1(speed_data)
  Measure distance/1(ultrasonic_sensor_data) -> Detect objects/3(ultrasonic_data)
  Bus Element In1/1 -> Acquire images/1(Obstacles)
  Bus Element In2/1 -> Emit laser impulse/1(Obstacles)
  Bus Element In3/1 -> Emit ultrasonic waves/2(Obstacles)
  Filtering/1(ObjectDetected) -> Bus Element Out1/1
  Bus Element In4/1 -> Emit ultrasonic waves/1(Power)
  Bus Element In5/1 -> Emit laser impulse/2(Power)
  Bus Element In6/1 -> Acquire images/2(Power)

== system FunctionalArchitectureProj/ Execute Parachute Deployment/Detect emergency ==
  Bus Element In1 : Inport  PortName=Critical Emergency
  Bus Element Out1 : Outport  PortName=alert_signal

== system FunctionalArchitectureProj/ Execute Parachute Deployment/Execute the parachute ==
  Bus Element In1 : Inport  PortName=Trigger _signal

== system FunctionalArchitectureProj/ Execute Parachute Deployment/Trigger the mechanism ==
  Bus Element In1 : Inport  PortName=alert_signal
  Bus Element Out1 : Outport  PortName=Trigger _signal

== system FunctionalArchitectureProj/Actuate propellers/Regulate speed of Propeller ==
  Bus Element In2 : Inport  PortName=Single Motor Voltage
  Bus Element In1 : Inport  Port=2  PortName=Target_Speed
  Bus Element Out2 : Outport  PortName=data

== system FunctionalArchitectureProj/Actuate propellers/Set Target speed of propellers ==
  Bus Element In1 : Inport  PortName=Propulsion Command
  Bus Element Out1 : Outport  PortName=Target_Speed

== system FunctionalArchitectureProj/Actuate propellers/Split the energy ==
  Bus Element In1 : Inport  PortName=Power
  Bus Element In2 : Inport  Port=2  PortName=data
  Bus Element Out1 : Outport  PortName=Single Motor Voltage

== system FunctionalArchitectureProj/Control the flight/Avoid the obstacle ==
  Bus Element In2 : Inport  PortName=ObstacleDetected
  Bus Element Out1 : Outport  PortName=Obstacle Position

== system FunctionalArchitectureProj/Control the flight/Change direction ==
  Bus Element In1 : Inport  PortName=DirectionSignal
  Bus Element Out1 : Outport  PortName=Propulsion Command

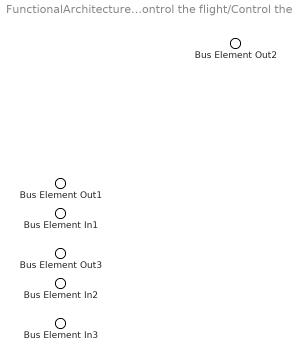
== system FunctionalArchitectureProj/Control the flight/Control the drone ==
  Bus Element In1 : Inport  PortName=Waypoint
  Bus Element In2 : Inport  Port=2  PortName=Drone_position
  Bus Element In3 : Inport  Port=3  PortName=Emergency Status
  Bus Element Out2 : Outport  PortName=Emergency_signal
  Bus Element Out1 : Outport  Port=2  PortName=Status
  Bus Element Out3 : Outport  Port=3  PortName=DirectionSignal

== system FunctionalArchitectureProj/Control the flight/Hover the drone ==
  Bus Element In1 : Inport  PortName=Emergency_signal
  Bus Element Out1 : Outport  PortName=Critical Emergenci
  Bus Element Out2 : Outport  Port=2  PortName=Emergency Status

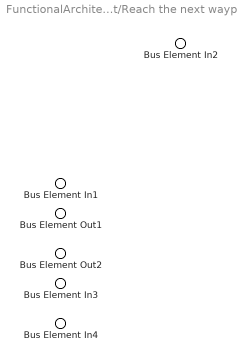
== system FunctionalArchitectureProj/Control the flight/Reach the next waypoint ==
  Bus Element In2 : Inport  PortName=Mission
  Bus Element In1 : Inport  Port=2  PortName=Drone Position
  Bus Element In3 : Inport  Port=3  PortName=Drone_speed
  Bus Element In4 : Inport  Port=4  PortName=Obstacle Position
  Bus Element Out1 : Outport  PortName=ActualPosition
  Bus Element Out2 : Outport  Port=2  PortName=Waypoint

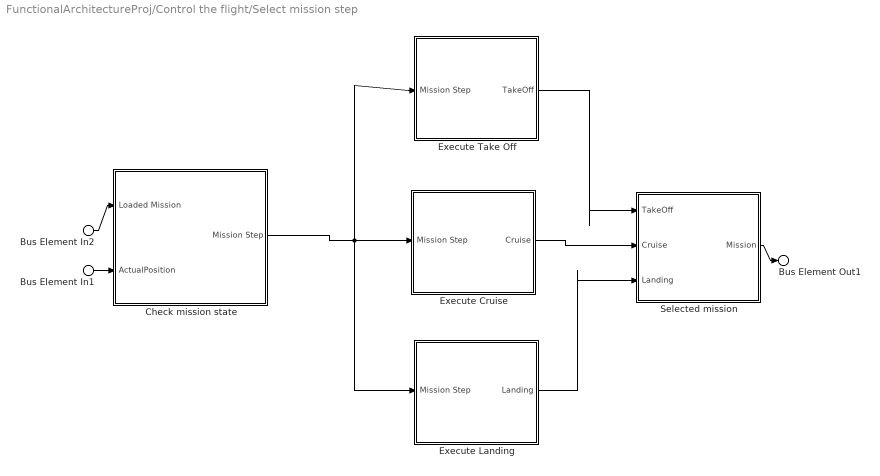
== system FunctionalArchitectureProj/Control the flight/Select mission step ==
  Bus Element In2 : Inport  PortName=Loaded Mission
  Bus Element In1 : Inport  Port=2  PortName=ActualPosition
  Check mission state : Subsystem
      settings: PortSchema="{\"entries\":[{\"content\":{\"headerSize\":26,\"margin\":15,\"minimumSpacing\":25,\"sides\":[{\"content\":{\"connectorIds\":[\"In1\",\"In2\"]},\"type\":\"ConnectorPlacement.EquallySpacedRectSide\",\"uuid\":\"ae43e0f9-cb81-4c7d-a5a1-6ddd261c3f36\"},{\"content\":{\"connectorIds\":[\"Out1\"],\"side\":\"RIGHT\"},\"type\":\"ConnectorPlacement.EquallySpacedRectSide\",\"uuid\":\"454013ea-826f-4879-bd33-a0fc10a3e69e\"},{\"content\":{\"connectorIds\":[],\"side\":\"TOP\"},\"type\":\"ConnectorPlacement.EquallySpacedRectSide\",\"uuid\":\"d045879a-9dfe-4c38-a274-6118b00e003b\"}]},\"type\":\"ConnectorPlacement.EquallySpacedConnector\",\"uuid\":\"e33c714e-0ae2-4a56-8ce0-f9b8de85daa2\"}],\"packageUris\":[\"http://schema.mathworks.com/mf0/Connector/R2020b\"],\"version\":\"1.0\"}"
  Execute Cruise : Subsystem
      settings: PortSchema="{\"entries\":[{\"content\":{\"headerSize\":26,\"margin\":15,\"minimumSpacing\":25,\"sides\":[{\"content\":{\"connectorIds\":[\"In1\"]},\"type\":\"ConnectorPlacement.EquallySpacedRectSide\",\"uuid\":\"ae43e0f9-cb81-4c7d-a5a1-6ddd261c3f36\"},{\"content\":{\"connectorIds\":[\"Out1\"],\"side\":\"RIGHT\"},\"type\":\"ConnectorPlacement.EquallySpacedRectSide\",\"uuid\":\"454013ea-826f-4879-bd33-a0fc10a3e69e\"},{\"content\":{\"connectorIds\":[],\"side\":\"TOP\"},\"type\":\"ConnectorPlacement.EquallySpacedRectSide\",\"uuid\":\"d045879a-9dfe-4c38-a274-6118b00e003b\"}]},\"type\":\"ConnectorPlacement.EquallySpacedConnector\",\"uuid\":\"e33c714e-0ae2-4a56-8ce0-f9b8de85daa2\"}],\"packageUris\":[\"http://schema.mathworks.com/mf0/Connector/R2020b\"],\"version\":\"1.0\"}"
  Execute Landing : Subsystem
      settings: PortSchema="{\"entries\":[{\"content\":{\"headerSize\":26,\"margin\":15,\"minimumSpacing\":25,\"sides\":[{\"content\":{\"connectorIds\":[\"In1\"]},\"type\":\"ConnectorPlacement.EquallySpacedRectSide\",\"uuid\":\"ae43e0f9-cb81-4c7d-a5a1-6ddd261c3f36\"},{\"content\":{\"connectorIds\":[\"Out1\"],\"side\":\"RIGHT\"},\"type\":\"ConnectorPlacement.EquallySpacedRectSide\",\"uuid\":\"454013ea-826f-4879-bd33-a0fc10a3e69e\"},{\"content\":{\"connectorIds\":[],\"side\":\"TOP\"},\"type\":\"ConnectorPlacement.EquallySpacedRectSide\",\"uuid\":\"d045879a-9dfe-4c38-a274-6118b00e003b\"}]},\"type\":\"ConnectorPlacement.EquallySpacedConnector\",\"uuid\":\"e33c714e-0ae2-4a56-8ce0-f9b8de85daa2\"}],\"packageUris\":[\"http://schema.mathworks.com/mf0/Connector/R2020b\"],\"version\":\"1.0\"}"
  Execute Take Off : Subsystem
      settings: PortSchema="{\"entries\":[{\"content\":{\"headerSize\":26,\"margin\":15,\"minimumSpacing\":25,\"sides\":[{\"content\":{\"connectorIds\":[\"In1\"]},\"type\":\"ConnectorPlacement.EquallySpacedRectSide\",\"uuid\":\"ae43e0f9-cb81-4c7d-a5a1-6ddd261c3f36\"},{\"content\":{\"connectorIds\":[\"Out1\"],\"side\":\"RIGHT\"},\"type\":\"ConnectorPlacement.EquallySpacedRectSide\",\"uuid\":\"454013ea-826f-4879-bd33-a0fc10a3e69e\"},{\"content\":{\"connectorIds\":[],\"side\":\"TOP\"},\"type\":\"ConnectorPlacement.EquallySpacedRectSide\",\"uuid\":\"d045879a-9dfe-4c38-a274-6118b00e003b\"}]},\"type\":\"ConnectorPlacement.EquallySpacedConnector\",\"uuid\":\"e33c714e-0ae2-4a56-8ce0-f9b8de85daa2\"}],\"packageUris\":[\"http://schema.mathworks.com/mf0/Connector/R2020b\"],\"version\":\"1.0\"}"
  Selected mission : Subsystem
      settings: PortSchema="{\"entries\":[{\"content\":{\"headerSize\":26,\"margin\":15,\"minimumSpacing\":25,\"sides\":[{\"content\":{\"connectorIds\":[\"In1\",\"In2\",\"In3\"]},\"type\":\"ConnectorPlacement.EquallySpacedRectSide\",\"uuid\":\"ae43e0f9-cb81-4c7d-a5a1-6ddd261c3f36\"},{\"content\":{\"connectorIds\":[\"Out1\"],\"side\":\"RIGHT\"},\"type\":\"ConnectorPlacement.EquallySpacedRectSide\",\"uuid\":\"454013ea-826f-4879-bd33-a0fc10a3e69e\"},{\"content\":{\"connectorIds\":[],\"side\":\"TOP\"},\"type\":\"ConnectorPlacement.EquallySpacedRectSide\",\"uuid\":\"d045879a-9dfe-4c38-a274-6118b00e003b\"}]},\"type\":\"ConnectorPlacement.EquallySpacedConnector\",\"uuid\":\"e33c714e-0ae2-4a56-8ce0-f9b8de85daa2\"}],\"packageUris\":[\"http://schema.mathworks.com/mf0/Connector/R2020b\"],\"version\":\"1.0\"}"
  Bus Element Out1 : Outport  PortName=Mission
  wires:
  Check mission state/1(Mission Step) -> Execute Take Off/1(Mission Step), Execute Landing/1(Mission Step), Execute Cruise/1(Mission Step)
  Bus Element In1/1 -> Check mission state/2(ActualPosition)
  Bus Element In2/1 -> Check mission state/1(Loaded Mission)
  Execute Take Off/1(TakeOff) -> Selected mission/1(TakeOff)
  Execute Cruise/1(Cruise) -> Selected mission/2(Cruise)
  Execute Landing/1(Landing) -> Selected mission/3(Landing)
  Selected mission/1(Mission) -> Bus Element Out1/1

== system FunctionalArchitectureProj/Deliver the payload/Acquisition data ==
  Bus Element In1 : Inport  PortName=Temperature_data
  Bus Element Out1 : Outport  PortName=Raw_Data

== system FunctionalArchitectureProj/Deliver the payload/Activate Fans ==
  Bus Element In1 : Inport  PortName=voltage2
  Bus Element Out1 : Outport  PortName=fans energy

== system FunctionalArchitectureProj/Deliver the payload/Communicate status ==
  Bus Element In1 : Inport  PortName=Status_open
  Bus Element In2 : Inport  Port=2  PortName=status_close
  Bus Element Out1 : Outport  PortName=Reed data

== system FunctionalArchitectureProj/Deliver the payload/Detect door status ==
  Bus Element In1 : Inport  PortName=Reed_data
  Ensure the status : Subsystem
      settings: PortSchema="{\"entries\":[{\"content\":{\"headerSize\":26,\"margin\":15,\"minimumSpacing\":25,\"sides\":[{\"content\":{\"connectorIds\":[\"In1\"]},\"type\":\"ConnectorPlacement.EquallySpacedRectSide\",\"uuid\":\"8049ad02-19ac-4f14-9b36-a42a8615a652\"},{\"content\":{\"connectorIds\":[\"Out1\",\"Out2\"],\"side\":\"RIGHT\"},\"type\":\"ConnectorPlacement.EquallySpacedRectSide\",\"uuid\":\"a3e2e02d-3567-418c-afac-b08313eb92f4\"},{\"content\":{\"side\":\"TOP\"},\"type\":\"ConnectorPlacement.EquallySpacedRectSide\",\"uuid\":\"0a99e400-62af-4ce6-9b2a-3ec4b8645f60\"},{\"content\":{\"side\":\"BOTTOM\"},\"type\":\"ConnectorPlacement.EquallySpacedRectSide\",\"uuid\":\"bf2e4bd0-f1ec-4cbb-9a7f-78e8e5ff900a\"}]},\"type\":\"ConnectorPlacement.EquallySpacedConnector\",\"uuid\":\"ada0285e-d286-47a3-bd64-ce4f3c6c3017\"}],\"packageUris\":[\"http://schema.mathworks.com/mf0/Connector/R2020b\"],\"version\":\"1.0\"}"
  Bus Element Out1 : Outport  PortName=Status_open
  Bus Element Out2 : Outport  Port=2  PortName=status_close
  wires:
  Ensure the status/1(YES) -> Bus Element Out1/1
  Ensure the status/2(NC) -> Bus Element Out2/1
  Bus Element In1/1 -> Ensure the status/1(Reed_data)

== system FunctionalArchitectureProj/Deliver the payload/Detect magnetic field ==
  Bus Element Out1 : Outport  PortName=Magnetize

== system FunctionalArchitectureProj/Deliver the payload/Make decision ==
  Bus Element In1 : Inport  PortName=Cooler data
  Bus Element Out1 : Outport  PortName=Alert_signal

== system FunctionalArchitectureProj/Deliver the payload/Monitor Temperature  ==
  Bus Element In2 : Inport  PortName=TemperatureOUT
  Bus Element In1 : Inport  Port=2  PortName=Power
  Bus Element Out1 : Outport  PortName=Temperature_data
  Bus Element Out2 : Outport  Port=2  PortName=voltage

== system FunctionalArchitectureProj/Deliver the payload/Process data ==
  Bus Element In1 : Inport  PortName=Raw_Data
  Bus Element Out1 : Outport  PortName=Processed_Data

== system FunctionalArchitectureProj/Deliver the payload/Receive Reed Sensor Signal ==
  Bus Element In1 : Inport  PortName=Power
  Bus Element In2 : Inport  Port=2  PortName=Magnetize
  Bus Element Out1 : Outport  PortName=Reed_Data

== system FunctionalArchitectureProj/Deliver the payload/Reduce heat ==
  Bus Element In1 : Inport  PortName=fans energy
  Bus Element Out1 : Outport  PortName=TemperatureIN

== system FunctionalArchitectureProj/Deliver the payload/Regulate cooler ==
  Bus Element In2 : Inport  PortName=voltage
  Bus Element In1 : Inport  Port=2  PortName=Processed_Data
  Bus Element Out2 : Outport  PortName=voltage1
  Bus Element Out1 : Outport  Port=2  PortName=Cooler data

== system FunctionalArchitectureProj/Deliver the payload/Trigger Cooling Mechanism ==
  Bus Element In2 : Inport  PortName=voltage1
  Bus Element In1 : Inport  Port=2  PortName=Alert_signal
  Bus Element Out1 : Outport  PortName=voltage2

== system FunctionalArchitectureProj/Manage Data Transmission /Decode signals ==
  Bus Element In1 : Inport  PortName=process data
  Bus Element Out1 : Outport  PortName=decoded data

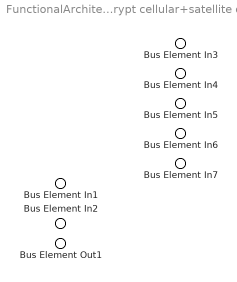
== system FunctionalArchitectureProj/Manage Data Transmission /Decrypt cellular+satellite data ==
  Bus Element In7 : Inport  PortName=Reed data
  Bus Element In5 : Inport  Port=2  PortName=COM_IN
  Bus Element In4 : Inport  Port=3  PortName=ControlStationIN
  Bus Element In3 : Inport  Port=4  PortName=Status
  Bus Element In6 : Inport  Port=5  PortName=TempContrIN
  Bus Element In1 : Inport  Port=6  PortName=Power
  Bus Element In2 : Inport  Port=7  PortName=UserIN
  Bus Element Out1 : Outport  PortName=data_decrypted

== system FunctionalArchitectureProj/Manage Data Transmission /Encode signals ==
  Bus Element In1 : Inport  PortName=raw data
  Bus Element Out1 : Outport  PortName=process data

== system FunctionalArchitectureProj/Manage Data Transmission /Encrypt data ==
  Bus Element In1 : Inport  PortName=signal
  Bus Element Out1 : Outport  PortName=encrypted data

== system FunctionalArchitectureProj/Manage Data Transmission /Establish connections ==
  Bus Element In1 : Inport  PortName=decoded data
  Bus Element Out1 : Outport  PortName=communication links

== system FunctionalArchitectureProj/Manage Data Transmission /Make decision ==
  Bus Element In2 : Inport  PortName=satellite
  Bus Element In1 : Inport  Port=2  PortName=cellular
  Bus Element Out1 : Outport  PortName=raw data

== system FunctionalArchitectureProj/Manage Data Transmission /Monitor signal strength ==
  Bus Element In1 : Inport  PortName=communication links
  Bus Element Out1 : Outport  PortName=signal

== system FunctionalArchitectureProj/Manage Data Transmission /Provide redundancy ==
  Bus Element In1 : Inport  PortName=encrypted data
  Bus Element Out4 : Outport  PortName=COM_OUT
  Bus Element Out3 : Outport  Port=2  PortName=UserOUT
  Bus Element Out2 : Outport  Port=3  PortName=ControlStationOut
  Bus Element Out1 : Outport  Port=4  PortName=TempContrOUT

== system FunctionalArchitectureProj/Manage Data Transmission /Receive data ==
  Bus Element In2 : Inport  PortName=data_decrypted
  Bus Element Out1 : Outport  PortName=data

== system FunctionalArchitectureProj/Manage Data Transmission /Switch networks ==
  Bus Element In1 : Inport  PortName=data1
  Bus Element Out1 : Outport  PortName=cellular
  Bus Element Out2 : Outport  Port=2  PortName=satellite

== system FunctionalArchitectureProj/Manage Data Transmission /Transmit data ==
  Bus Element In1 : Inport  PortName=data1
  Bus Element Out1 : Outport  PortName=data 1

== system FunctionalArchitectureProj/Navigate the environment/Check changing in airspeed ==
  Bus Element In1 : Inport  PortName=critical_airspeed_data
  Bus Element Out1 : Outport  PortName=changing_airspeed
